simulink model "wlan_phy_tx_pmd"  (Simulink 7.8)
settings: Solver=VariableStepDiscrete  SolverMode=SingleTasking  StartTime=0.0  StopTime=inf  RelTol=1e-3
PostLoadFcn:
  | wlan_phy_tx_init
InitFcn:
  | wlan_phy_tx_init
StartFcn:
  | wlan_phy_tx_init
undefined symbols (not defined in the file): gcbh, ht_preamble_rom, MAX_CP_LEN, MAX_DATA_BITS_PER_SYM_PERIOD, MAX_NCBPS, MAX_NUM_BYTES, MAX_NUM_SC, MAX_NUM_SYMS, mcs_rom_11ag, mcs_rom_11n, Mod_Constellation_16QAM, Mod_Constellation_64QAM, Mod_Constellation_BPSK, Mod_Constellation_QPSK, Preamble_IQ, Preamble_IQ_scaled, tx_sim, wlan_tx_interleave_rom, xlBlockLoadCallback, xlGetNormalizedPeriod
libraries: xbsIndex_r4 x1358, xbsEDKLib_r4 x1
(part 6 of 10)

== system wlan_phy_tx_pmd/Start Ctrl/Simulation Stop ==
  TX_DONE : Inport
  Constant1 : Constant  Value=tx_sim.num_pkts
  Counter : xbsIndex_r4/Counter  cnt_type=Free Running  cnt_to=Inf  operation=Up  start_count=0  cnt_by_val=1  arith_type=Unsigned  n_bits=8  bin_pt=0  load_pin=off  rst=off  en=on  explicit_period=off  period=1  dbl_ovrd=off  use_behavioral_HDL=off  implementation=Fabric  block_type=counter
  Delay : xbsIndex_r4/Delay  rst=off  infoeditControl=Selection of Reset will increase slice count due to use of real FFs and instead of SRLs  en=off  latency=500  dbl_ovrd=off  reg_retiming=off  block_type=delay
  Delay1 : xbsIndex_r4/Delay  rst=off  infoeditControl=Selection of Reset will increase slice count due to use of real FFs and instead of SRLs  en=off  latency=32  dbl_ovrd=off  reg_retiming=off  block_type=delay
  Delay2 : Delay  DelayLength=400  SampleTime=1
  Disregard Subsystem : xbsIndex_r4/Disregard Subsystem  Tag=discardX  block_type=disregard
  Gateway Out{1..4} (4 alike) : xbsIndex_r4/Gateway Out  inherit_from_input=off  hdl_port=off  timing_constraint=None  locs_specified=off  LOCs={}  UseAsDAC=off  DACChannel='1'  block_type=gatewayout
  Posedge3 : Subsystem
  Radio TxEn-RxEn : Scope  NumInputPorts=7
      settings: TimeRange=14000  YMin=-1~2~-1~-1~-1~-1~-1  YMax=1~2~1~1~1~1~1  SaveName=ScopeData14
  Relational Operator : RelationalOperator  OutDataTypeStr=boolean
  S-R Latch1 : Subsystem
  Stop Simulation : Stop
  tag scope: sim_Start_New_Tx=global
  wires:
  Posedge3/1(Q) -> Counter/1, Delay/1
  Counter/1 -> Gateway Out1/1, Gateway Out4/1
  Constant1/1 -> Relational Operator/2
  Relational Operator/1 -> Delay2/1
  Gateway Out1/1 -> Relational Operator/1
  TX_DONE/1 -> Posedge3/1(D), Gateway Out3/1
  Delay2/1 -> Stop Simulation/1, Radio TxEn-RxEn/3  "Stop"
  S-R Latch1/1(Q) -> Delay1/1, Gateway Out2/1  "Start"
  Gateway Out3/1 -> Radio TxEn-RxEn/1  "TX_DONE"
  Gateway Out4/1 -> Radio TxEn-RxEn/2  "Pkt Count"
  Delay/1 -> S-R Latch1/1(S)
  Delay1/1 -> S-R Latch1/2(R)
  Gateway Out2/1 -> [sim_Start_New_Tx], Radio TxEn-RxEn/4  "Start"

== system wlan_phy_tx_pmd/Start Ctrl/Tx Active Debug Signal ==
  note: TX_RUNNING is a debug signal usually tied to an FPGA
      | output for real-time observation on an oscilloscope. The mux
      | here selects between the raw Tx Active signal or
      | a delayed version. The raw signal is useful for observing
      | MAC timing. The delayed version is useful for triggering
      | packet detection at an Rx node.
  Tx Active : Inport
  Convert9 : xbsIndex_r4/Convert  gui_display_data_type=Fixed-point  arith_type=Unsigned  n_bits=1  bin_pt=0  float_type=Single  exp_bits=8  fraction_bits=24  quantization=Truncate  overflow=Wrap  en=off  latency=0  dbl_ovrd=off  pipeline=off  block_type=convert
  Dly : Subsystem
  Mux : xbsIndex_r4/Mux  inputs=2  en=off  latency=0  precision=Full  arith_type=Unsigned  n_bits=16  bin_pt=14  quantization=Truncate  overflow=Wrap  dbl_ovrd=off  block_type=mux
  Register : xbsIndex_r4/Register  init=0  rst=off  en=off  dbl_ovrd=off  block_type=register
  Register1 : xbsIndex_r4/Register  init=0  rst=off  en=off  dbl_ovrd=off  block_type=register
  Register5 : xbsIndex_r4/Register  init=0  rst=off  en=off  dbl_ovrd=off  block_type=register
  dbg_TX_RUNNING : xbsIndex_r4/Gateway Out  inherit_from_input=off  hdl_port=on  timing_constraint=None  locs_specified=off  LOCs={}  UseAsDAC=off  DACChannel='1'  block_type=gatewayout
  wires:
  Register/1 -> Register1/1
  Register1/1 -> dbg_TX_RUNNING/1
  Dly/1(Q) -> Mux/3
  [regTx_TxRunning_Output_Sel] -> Mux/1
  Mux/1 -> Register/1
  Register5/1 -> Dly/1(D), Convert9/1
  Convert9/1 -> Mux/2
  Tx Active/1 -> Register5/1

== system wlan_phy_tx_pmd/Start Ctrl/Tx Gain ==
  note: Pass through MAC Tx gain setting to radio controller
  Sw Tx : Inport
  Hw Tx : Inport  Port=2
  Convert : xbsIndex_r4/Convert  gui_display_data_type=Boolean  arith_type=Boolean  n_bits=16  bin_pt=14  float_type=Single  exp_bits=8  fraction_bits=24  quantization=Truncate  overflow=Wrap  en=off  latency=0  dbl_ovrd=off  pipeline=off  block_type=convert
  Convert1 : xbsIndex_r4/Convert  gui_display_data_type=Boolean  arith_type=Boolean  n_bits=16  bin_pt=14  float_type=Single  exp_bits=8  fraction_bits=24  quantization=Truncate  overflow=Wrap  en=off  latency=0  dbl_ovrd=off  pipeline=off  block_type=convert
  Logical1 : xbsIndex_r4/Logical  logical_function=OR  inputs=2  en=off  latency=0  precision=Full  arith_type=Unsigned  n_bits=16  bin_pt=0  align_bp=on  dbl_ovrd=off  block_type=logical
  PHY_TX_GAIN_A : xbsIndex_r4/Gateway In  gui_display_data_type=Fixed-point  arith_type=Unsigned  n_bits=6  bin_pt=0  preci_type=Single  exp_width=8  frac_width=24  quantization="Round  (unbiased: +/- Inf)"  overflow=Saturate  period=1  dbl_ovrd=off  timing_constraint=None  locs_specified=off  LOCs={}  UseAsADC=off  ADCChannel='1'  inherit_from_input=off  hdl_port=on  block_type=gatewayin
  PHY_TX_GAIN_B : xbsIndex_r4/Gateway In  gui_display_data_type=Fixed-point  arith_type=Unsigned  n_bits=6  bin_pt=0  preci_type=Single  exp_width=8  frac_width=24  quantization="Round  (unbiased: +/- Inf)"  overflow=Saturate  period=1  dbl_ovrd=off  timing_constraint=None  locs_specified=off  LOCs={}  UseAsADC=off  ADCChannel='1'  inherit_from_input=off  hdl_port=on  block_type=gatewayin
  PHY_TX_GAIN_C : xbsIndex_r4/Gateway In  gui_display_data_type=Fixed-point  arith_type=Unsigned  n_bits=6  bin_pt=0  preci_type=Single  exp_width=8  frac_width=24  quantization="Round  (unbiased: +/- Inf)"  overflow=Saturate  period=1  dbl_ovrd=off  timing_constraint=None  locs_specified=off  LOCs={}  UseAsADC=off  ADCChannel='1'  inherit_from_input=off  hdl_port=on  block_type=gatewayin
  PHY_TX_GAIN_D : xbsIndex_r4/Gateway In  gui_display_data_type=Fixed-point  arith_type=Unsigned  n_bits=6  bin_pt=0  preci_type=Single  exp_width=8  frac_width=24  quantization="Round  (unbiased: +/- Inf)"  overflow=Saturate  period=1  dbl_ovrd=off  timing_constraint=None  locs_specified=off  LOCs={}  UseAsADC=off  ADCChannel='1'  inherit_from_input=off  hdl_port=on  block_type=gatewayin
  Register{1,3,5,7} (4 alike) : xbsIndex_r4/Register  init=0  rst=off  en=off  dbl_ovrd=off  block_type=register
  Register{2,4,6,8} (4 alike) : xbsIndex_r4/Register  init=0  rst=off  en=on  dbl_ovrd=off  block_type=register
      settings: xl_area=[1 1 0 0 0 0 0]  block_version=VER_STRING_GOES_HERE
  Tx Gain A : Outport
  Tx Gain B : Outport  Port=2
  Tx Gain C : Outport  Port=3
  Tx Gain D : Outport  Port=4
  wires:
  Convert1/1 -> Logical1/2
  Hw Tx/1 -> Convert1/1
  Sw Tx/1 -> Convert/1
  PHY_TX_GAIN_A/1 -> Register2/1
  Convert/1 -> Logical1/1
  Register2/1 -> Register1/1
  Logical1/1 -> Register2/2, Register4/2, Register6/2, Register8/2
  Register1/1 -> Tx Gain A/1
  Register4/1 -> Register3/1
  Register3/1 -> Tx Gain B/1
  PHY_TX_GAIN_B/1 -> Register4/1
  Register6/1 -> Register5/1
  Register5/1 -> Tx Gain C/1
  Register8/1 -> Register7/1
  Register7/1 -> Tx Gain D/1
  PHY_TX_GAIN_C/1 -> Register6/1
  PHY_TX_GAIN_D/1 -> Register8/1

== system wlan_phy_tx_pmd/Start Ctrl/negedge ==
  D : Inport
  Delay : xbsIndex_r4/Delay  rst=off  infoeditControl=Selection of Reset will increase slice count due to use of real FFs and instead of SRLs  en=off  latency=1  dbl_ovrd=off  reg_retiming=off  block_type=delay
      settings: infoedit=Hardware notes: A delay line is a chain, each link of which is an SRL16 followed by a flip-flop. If register retiming is enabled, the delay line is a chain of flip-flops.  xl_area=[1 1 0 0 0 0 0]  block_version=VER_STRING_GOES_HERE
  Inverter : xbsIndex_r4/Inverter  en=off  latency=0  dbl_ovrd=off  block_type=inv
      settings: xl_area=[0 0 0 0 0 0 0]  block_version=VER_STRING_GOES_HERE
  Logical1 : xbsIndex_r4/Logical  logical_function=AND  inputs=2  en=off  latency=0  precision=Full  arith_type=Unsigned  n_bits=8  bin_pt=2  align_bp=on  dbl_ovrd=off  block_type=logical
      settings: xl_area=[1 0 0 1 0 0 0]  block_version=VER_STRING_GOES_HERE
  Q : Outport
  wires:
  D/1 -> Delay/1, Inverter/1
  Logical1/1 -> Q/1
  Delay/1 -> Logical1/1
  Inverter/1 -> Logical1/2

== system wlan_phy_tx_pmd/IFFT and Cyclic Prefix/Buffer and Cyclic Prefix/Control ==
  note: Hacky way to skip last cycle of counter. Avoids
      | having to compute SC+CP-1.
  tlast : Inport
  AddSub : xbsIndex_r4/AddSub  mode=Addition  use_carryin=off  use_carryout=off  en=off  latency=1  precision=Full  arith_type=Unsigned  n_bits=16  bin_pt=14  quantization=Truncate  overflow=Wrap  dbl_ovrd=off  use_behavioral_HDL=off  hw_selection=Fabric  pipelined=off  block_type=addsub
  Counter : xbsIndex_r4/Counter  cnt_type=Free Running  cnt_to=47  operation=Up  start_count=0  cnt_by_val=1  arith_type=Unsigned  n_bits=ceil(log2(MAX_NUM_SC + MAX_CP_LEN) + 1)  bin_pt=0  load_pin=off  rst=on  en=on  explicit_period=off  period=1  dbl_ovrd=off  use_behavioral_HDL=off  implementation=Fabric  block_type=counter
  Inverter1 : xbsIndex_r4/Inverter  en=off  latency=0  dbl_ovrd=off  block_type=inv
      settings: xl_area=[0 0 0 0 0 0 0]  block_version=VER_STRING_GOES_HERE
  Inverter2 : xbsIndex_r4/Inverter  en=off  latency=0  dbl_ovrd=off  block_type=inv
      settings: xl_area=[0 0 0 0 0 0 0]  block_version=VER_STRING_GOES_HERE
  Logical2 : xbsIndex_r4/Logical  logical_function=AND  inputs=2  en=off  latency=0  precision=Full  arith_type=Unsigned  n_bits=16  bin_pt=0  align_bp=on  dbl_ovrd=off  block_type=logical
  Relational3 : xbsIndex_r4/Relational  mode=a>=b  en=off  latency=0  dbl_ovrd=off  block_type=relational
  S-R Latch1 : Subsystem
  Rd Addr : Outport
  Valid : Outport  Port=2
  wires:
  [regTx_NUM_SC] -> AddSub/1
  Inverter1/1 -> Counter/1
  S-R Latch1/1(Q) -> Counter/2, Inverter1/1, Logical2/1
  Counter/1 -> Relational3/1, Rd Addr/1
  [regTx_CP_LEN] -> AddSub/2
  Relational3/1 -> S-R Latch1/2(R), Inverter2/1
  Inverter2/1 -> Logical2/2
  tlast/1 -> S-R Latch1/1(S)
  Logical2/1 -> Valid/1
  AddSub/1 -> Relational3/2

== system wlan_phy_tx_pmd/IFFT and Cyclic Prefix/Buffer and Cyclic Prefix/I/Q Concat ==
  I : Inport
  Q : Inport  Port=2
  Concat : xbsIndex_r4/Concat  num_inputs=2  dbl_ovrd=off  block_type=concat
  Reinterpret : xbsIndex_r4/Reinterpret  force_arith_type=on  arith_type=Unsigned  force_bin_pt=on  bin_pt=0  block_type=reinterpret
  Reinterpret1 : xbsIndex_r4/Reinterpret  force_arith_type=on  arith_type=Unsigned  force_bin_pt=on  bin_pt=0  block_type=reinterpret
  IQ : Outport
  wires:
  Reinterpret/1 -> Concat/1
  Reinterpret1/1 -> Concat/2
  I/1 -> Reinterpret/1
  Concat/1 -> IQ/1
  Q/1 -> Reinterpret1/1

== system wlan_phy_tx_pmd/IFFT and Cyclic Prefix/Buffer and Cyclic Prefix/I/Q Slice ==
  IQ : Inport
  Reinterpret2 : xbsIndex_r4/Reinterpret  force_arith_type=on  arith_type="Signed  (2's comp)"  force_bin_pt=on  bin_pt=15  block_type=reinterpret
  Reinterpret3 : xbsIndex_r4/Reinterpret  force_arith_type=on  arith_type="Signed  (2's comp)"  force_bin_pt=on  bin_pt=15  block_type=reinterpret
  Slice : xbsIndex_r4/Slice  nbits=16  boolean_output=off  mode=Upper Bit Location + Width  bit1=0  base1=MSB of Input  bit0=0  base0=LSB of Input  dbl_ovrd=off  block_type=slice
  Slice1 : xbsIndex_r4/Slice  nbits=16  boolean_output=off  mode=Lower Bit Location + Width  bit1=0  base1=MSB of Input  bit0=0  base0=LSB of Input  dbl_ovrd=off  block_type=slice
  I : Outport
  Q : Outport  Port=2
  wires:
  Reinterpret3/1 -> Q/1
  Reinterpret2/1 -> I/1
  IQ/1 -> Slice/1, Slice1/1
  Slice1/1 -> Reinterpret3/1
  Slice/1 -> Reinterpret2/1

== system wlan_phy_tx_pmd/IFFT and Cyclic Prefix/FIFO/I/Q Concat ==
  I : Inport
  Q : Inport  Port=2
  Concat : xbsIndex_r4/Concat  num_inputs=2  dbl_ovrd=off  block_type=concat
  Reinterpret : xbsIndex_r4/Reinterpret  force_arith_type=on  arith_type=Unsigned  force_bin_pt=on  bin_pt=0  block_type=reinterpret
  Reinterpret1 : xbsIndex_r4/Reinterpret  force_arith_type=on  arith_type=Unsigned  force_bin_pt=on  bin_pt=0  block_type=reinterpret
  IQ : Outport
  wires:
  Reinterpret/1 -> Concat/1
  Reinterpret1/1 -> Concat/2
  I/1 -> Reinterpret/1
  Concat/1 -> IQ/1
  Q/1 -> Reinterpret1/1

== system wlan_phy_tx_pmd/IFFT and Cyclic Prefix/FIFO/I/Q Slice ==
  IQ : Inport
  Reinterpret2 : xbsIndex_r4/Reinterpret  force_arith_type=on  arith_type="Signed  (2's comp)"  force_bin_pt=on  bin_pt=15  block_type=reinterpret
  Reinterpret3 : xbsIndex_r4/Reinterpret  force_arith_type=on  arith_type="Signed  (2's comp)"  force_bin_pt=on  bin_pt=15  block_type=reinterpret
  Slice : xbsIndex_r4/Slice  nbits=16  boolean_output=off  mode=Upper Bit Location + Width  bit1=0  base1=MSB of Input  bit0=0  base0=LSB of Input  dbl_ovrd=off  block_type=slice
  Slice1 : xbsIndex_r4/Slice  nbits=16  boolean_output=off  mode=Lower Bit Location + Width  bit1=0  base1=MSB of Input  bit0=0  base0=LSB of Input  dbl_ovrd=off  block_type=slice
  I : Outport
  Q : Outport  Port=2
  wires:
  Reinterpret3/1 -> Q/1
  Reinterpret2/1 -> I/1
  IQ/1 -> Slice/1, Slice1/1
  Slice1/1 -> Reinterpret3/1
  Slice/1 -> Reinterpret2/1

== system wlan_phy_tx_pmd/OFDM Symbol Ctrl/Sym Counter/S-R Latch1 ==
  S : Inport
  R : Inport  Port=2
  Constant1 : xbsIndex_r4/Constant  const=1  gui_display_data_type=Fixed-point  arith_type=Boolean  n_bits=1  bin_pt=0  preci_type=Single  exp_width=8  frac_width=24  explicit_period=off  period=1  equ=P=C  opselect=C  inp2=PCIN>>17  opr=+  inp1=P  carry=CIN  dbl_ovrd=off  block_type=constant
      settings: block_version=VER_STRING_GOES_HERE
  Convert1 : xbsIndex_r4/Convert  gui_display_data_type=Boolean  arith_type=Boolean  n_bits=1  bin_pt=0  float_type=Single  exp_bits=8  fraction_bits=24  quantization=Truncate  overflow=Wrap  en=off  latency=0  dbl_ovrd=off  pipeline=off  block_type=convert
  Convert2 : xbsIndex_r4/Convert  gui_display_data_type=Boolean  arith_type=Boolean  n_bits=1  bin_pt=0  float_type=Single  exp_bits=8  fraction_bits=24  quantization=Truncate  overflow=Wrap  en=off  latency=0  dbl_ovrd=off  pipeline=off  block_type=convert
  Register2 : xbsIndex_r4/Register  init=0  rst=on  en=on  dbl_ovrd=off  block_type=register
      settings: xl_area=[1 1 0 0 0 0 0]  block_version=VER_STRING_GOES_HERE
  Q : Outport
  wires:
  Convert2/1 -> Register2/3
  Convert1/1 -> Register2/2
  Constant1/1 -> Register2/1
  R/1 -> Convert1/1
  Register2/1 -> Q/1
  S/1 -> Convert2/1

== system wlan_phy_tx_pmd/OFDM Symbol Ctrl/Sym Samp Counter/Posedge1 ==
  D : Inport
  Delay : xbsIndex_r4/Delay  rst=off  infoeditControl=Selection of Reset will increase slice count due to use of real FFs and instead of SRLs  en=off  latency=1  dbl_ovrd=off  reg_retiming=off  block_type=delay
      settings: infoedit=Hardware notes: A delay line is a chain, each link of which is an SRL16 followed by a flip-flop. If register retiming is enabled, the delay line is a chain of flip-flops.  xl_area=[1 1 0 0 0 0 0]  block_version=VER_STRING_GOES_HERE
  Inverter : xbsIndex_r4/Inverter  en=off  latency=0  dbl_ovrd=off  block_type=inv
      settings: xl_area=[0 0 0 0 0 0 0]  block_version=VER_STRING_GOES_HERE
  Logical1 : xbsIndex_r4/Logical  logical_function=AND  inputs=2  en=off  latency=0  precision=Full  arith_type=Unsigned  n_bits=8  bin_pt=2  align_bp=on  dbl_ovrd=off  block_type=logical
      settings: xl_area=[1 0 0 1 0 0 0]  block_version=VER_STRING_GOES_HERE
  Q : Outport
  wires:
  Inverter/1 -> Logical1/1
  D/1 -> Logical1/2, Delay/1
  Logical1/1 -> Q/1
  Delay/1 -> Inverter/1

== system wlan_phy_tx_pmd/OFDM Symbol Ctrl/Sym Samp Counter/Posedge2 ==
  D : Inport
  Delay : xbsIndex_r4/Delay  rst=off  infoeditControl=Selection of Reset will increase slice count due to use of real FFs and instead of SRLs  en=off  latency=1  dbl_ovrd=off  reg_retiming=off  block_type=delay
      settings: infoedit=Hardware notes: A delay line is a chain, each link of which is an SRL16 followed by a flip-flop. If register retiming is enabled, the delay line is a chain of flip-flops.  xl_area=[1 1 0 0 0 0 0]  block_version=VER_STRING_GOES_HERE
  Inverter : xbsIndex_r4/Inverter  en=off  latency=0  dbl_ovrd=off  block_type=inv
      settings: xl_area=[0 0 0 0 0 0 0]  block_version=VER_STRING_GOES_HERE
  Logical1 : xbsIndex_r4/Logical  logical_function=AND  inputs=2  en=off  latency=0  precision=Full  arith_type=Unsigned  n_bits=8  bin_pt=2  align_bp=on  dbl_ovrd=off  block_type=logical
      settings: xl_area=[1 0 0 1 0 0 0]  block_version=VER_STRING_GOES_HERE
  Q : Outport
  wires:
  Delay/1 -> Inverter/1
  Logical1/1 -> Q/1
  D/1 -> Delay/1, Logical1/2
  Inverter/1 -> Logical1/1

== system wlan_phy_tx_pmd/OFDM Symbol Ctrl/Sym Samp Counter/S-R Latch2 ==
  S : Inport
  R : Inport  Port=2
  Constant1 : xbsIndex_r4/Constant  const=1  gui_display_data_type=Fixed-point  arith_type=Boolean  n_bits=1  bin_pt=0  preci_type=Single  exp_width=8  frac_width=24  explicit_period=off  period=1  equ=P=C  opselect=C  inp2=PCIN>>17  opr=+  inp1=P  carry=CIN  dbl_ovrd=off  block_type=constant
      settings: block_version=VER_STRING_GOES_HERE
  Convert1 : xbsIndex_r4/Convert  gui_display_data_type=Boolean  arith_type=Boolean  n_bits=1  bin_pt=0  float_type=Single  exp_bits=8  fraction_bits=24  quantization=Truncate  overflow=Wrap  en=off  latency=0  dbl_ovrd=off  pipeline=off  block_type=convert
  Convert2 : xbsIndex_r4/Convert  gui_display_data_type=Boolean  arith_type=Boolean  n_bits=1  bin_pt=0  float_type=Single  exp_bits=8  fraction_bits=24  quantization=Truncate  overflow=Wrap  en=off  latency=0  dbl_ovrd=off  pipeline=off  block_type=convert
  Register2 : xbsIndex_r4/Register  init=0  rst=on  en=on  dbl_ovrd=off  block_type=register
      settings: xl_area=[1 1 0 0 0 0 0]  block_version=VER_STRING_GOES_HERE
  Q : Outport
  wires:
  S/1 -> Convert2/1
  Register2/1 -> Q/1
  R/1 -> Convert1/1
  Constant1/1 -> Register2/1
  Convert1/1 -> Register2/2
  Convert2/1 -> Register2/3

== system wlan_phy_tx_pmd/PSDU Syms Gen/Index Gen/Bit Index Gen ==
  Bit Rd En : Inport
  Bit counter : xbsIndex_r4/Counter  cnt_type=Free Running  cnt_to=6  operation=Up  start_count=0  cnt_by_val=1  arith_type=Unsigned  n_bits=ceil(log2(MAX_NUM_BYTES))+3  bin_pt=0  load_pin=off  rst=on  en=on  explicit_period=off  period=1  dbl_ovrd=off  use_behavioral_HDL=off  implementation=Fabric  block_type=counter
  Bit in Byte : xbsIndex_r4/Slice  nbits=3  boolean_output=off  mode=Lower Bit Location + Width  bit1=0  base1=MSB of Input  bit0=0  base0=LSB of Input  dbl_ovrd=off  block_type=slice
      settings: block_version=8.2.02
  Bytes : xbsIndex_r4/Slice  nbits=ceil(log2(MAX_NUM_BYTES))  boolean_output=off  mode=Upper Bit Location + Width  bit1=0  base1=MSB of Input  bit0=0  base0=LSB of Input  dbl_ovrd=off  block_type=slice
      settings: block_version=8.2.02
  Constant3 : xbsIndex_r4/Constant  const=0  gui_display_data_type=Fixed-point  arith_type=Unsigned  n_bits=2  bin_pt=0  preci_type=Single  exp_width=8  frac_width=24  explicit_period=off  period=1  equ=P=C  opselect=C  inp2=PCIN>>17  opr=+  inp1=P  carry=CIN  dbl_ovrd=off  block_type=constant
      settings: block_version=VER_STRING_GOES_HERE
  Logical5 : xbsIndex_r4/Logical  logical_function=AND  inputs=2  en=off  latency=0  precision=Full  arith_type=Unsigned  n_bits=16  bin_pt=0  align_bp=on  dbl_ovrd=off  block_type=logical
  Relational1 : xbsIndex_r4/Relational  mode=a=b  en=off  latency=0  dbl_ovrd=off  block_type=relational
  Byte Ind : Outport
  Byte Ind Valid : Outport  Port=2
  Bit Sel : Outport  Port=3
  Bit Sel Valid : Outport  Port=4
  wires:
  Bit counter/1 -> Bytes/1, Bit in Byte/1
  Bit in Byte/1 -> Bit Sel/1, Relational1/1
  Bytes/1 -> Byte Ind/1
  Constant3/1 -> Relational1/2
  Relational1/1 -> Logical5/1
  Logical5/1 -> Byte Ind Valid/1
  Bit Rd En/1 -> Logical5/2, Bit Sel Valid/1, Bit counter/2
  [TX_RESET] -> Bit counter/1

== system wlan_phy_tx_pmd/PSDU Syms Gen/Index Gen/Bits Per Sym ==
  note: SIGNAL and HT-SIG sybmols always
      | contain 24 data bits (48 subcarriers, BPSK, 1/2 rate)
      | This mux selects the N_DBPS value for the current
      | MCS sometime after the SIGNAL (11a) or HT-SIG (11n)
      | fields are decoded.
      | Initial vlaue of N_DBPS register at mux in 0 must be non-zero!
  note: This block asserts the "Bit Rd En" output for a number of cycles
      | equal to the number of bits that will be read from the packet
      | buffer. Each OFDM symbol contains either 24 bits (for PHY
      | preamble symbols) or DATA_N_DBPS bits (set by the packet's MCS).
  Start : Inport
  Base Rate : Inport  Port=2
  Full Rate : Inport  Port=3
  Constant2 : xbsIndex_r4/Constant  const=24  gui_display_data_type=Fixed-point  arith_type=Unsigned  n_bits=5  bin_pt=0  preci_type=Single  exp_width=8  frac_width=24  explicit_period=off  period=1  equ=P=C  opselect=C  inp2=PCIN>>17  opr=+  inp1=P  carry=CIN  dbl_ovrd=off  block_type=constant
  Counter : xbsIndex_r4/Counter  cnt_type=Free Running  cnt_to=47  operation=Up  start_count=0  cnt_by_val=1  arith_type=Unsigned  n_bits=ceil(log2(MAX_DATA_BITS_PER_SYM_PERIOD))  bin_pt=0  load_pin=off  rst=on  en=on  explicit_period=off  period=1  dbl_ovrd=off  use_behavioral_HDL=off  implementation=Fabric  block_type=counter
  Inverter : xbsIndex_r4/Inverter  en=off  latency=0  dbl_ovrd=off  block_type=inv
      settings: xl_area=[0 0 0 0 0 0 0]  block_version=VER_STRING_GOES_HERE
  Inverter1 : xbsIndex_r4/Inverter  en=off  latency=0  dbl_ovrd=off  block_type=inv
      settings: xl_area=[0 0 0 0 0 0 0]  block_version=VER_STRING_GOES_HERE
  Logical1 : xbsIndex_r4/Logical  logical_function=OR  inputs=2  en=off  latency=0  precision=Full  arith_type=Unsigned  n_bits=8  bin_pt=2  align_bp=on  dbl_ovrd=off  block_type=logical
      settings: xl_area=[1 0 0 1 0 0 0]  block_version=VER_STRING_GOES_HERE
  Logical2 : xbsIndex_r4/Logical  logical_function=OR  inputs=2  en=off  latency=0  precision=Full  arith_type=Unsigned  n_bits=8  bin_pt=2  align_bp=on  dbl_ovrd=off  block_type=logical
      settings: xl_area=[1 0 0 1 0 0 0]  block_version=VER_STRING_GOES_HERE
  Logical3 : xbsIndex_r4/Logical  logical_function=AND  inputs=2  en=off  latency=0  precision=Full  arith_type=Unsigned  n_bits=8  bin_pt=2  align_bp=on  dbl_ovrd=off  block_type=logical
      settings: xl_area=[1 0 0 1 0 0 0]  block_version=VER_STRING_GOES_HERE
  Logical4 : xbsIndex_r4/Logical  logical_function=AND  inputs=2  en=off  latency=0  precision=Full  arith_type=Unsigned  n_bits=8  bin_pt=2  align_bp=on  dbl_ovrd=off  block_type=logical
      settings: xl_area=[1 0 0 1 0 0 0]  block_version=VER_STRING_GOES_HERE
  Mux : xbsIndex_r4/Mux  inputs=2  en=off  latency=0  precision=Full  arith_type=Unsigned  n_bits=16  bin_pt=14  quantization=Truncate  overflow=Wrap  dbl_ovrd=off  block_type=mux
  Register2 : xbsIndex_r4/Register  init=24  rst=on  en=on  dbl_ovrd=off  block_type=register
      settings: xl_area=[1 1 0 0 0 0 0]  block_version=VER_STRING_GOES_HERE
  Register3 : xbsIndex_r4/Register  init=0  rst=on  en=on  dbl_ovrd=off  block_type=register
      settings: xl_area=[1 1 0 0 0 0 0]  block_version=VER_STRING_GOES_HERE
  Relational3 : xbsIndex_r4/Relational  mode=a<b  en=off  latency=0  dbl_ovrd=off  block_type=relational
  S-R Latch1 : Subsystem
  Rd En : Outport
  wires:
  Logical2/1 -> Logical3/2
  Constant2/1 -> Mux/3
  Register2/1 -> Mux/2
  Register3/1 -> Mux/1
  [TX_RESET] -> Register3/2, Register2/2
  Inverter/1 -> Logical1/2
  Logical1/1 -> S-R Latch1/2(R)
  [TX_RESET] -> Logical1/1
  [OFDM_TX_DATA_N_DBPS] -> Register2/1
  Inverter1/1 -> Counter/1
  Relational3/1 -> Logical4/1, Inverter/1
  Mux/1 -> Relational3/2
  Counter/1 -> Relational3/1
  Logical3/1 -> Register3/3, Register2/3, S-R Latch1/1(S)
  S-R Latch1/1(Q) -> Logical4/2, Inverter1/1, Counter/2
  Logical4/1 -> Rd En/1
  Start/1 -> Logical3/1
  Base Rate/1 -> Logical2/2, Register3/1
  Full Rate/1 -> Logical2/1

== system wlan_phy_tx_pmd/PSDU Syms Gen/Modulate/16QAM Mod ==
  note: 16-QAM Bit Mapping:
      | [b0 b1] / [b2 b3]:
      | 00 = -3
      | 01 = -1
      | 11 = +1
      | 10 = +3
      | Norm = 1/sqrt(10)
  note: 00 -> 00
  note: 10 -> 01
  note: 01 -> 10
  note: 11 -> 11
  b[3:0] : Inport
  Constant1 : xbsIndex_r4/Constant  const=Mod_Constellation_16QAM(3)  gui_display_data_type=Fixed-point  arith_type=Signed (2's comp)  n_bits=12  bin_pt=11  preci_type=Single  exp_width=8  frac_width=24  explicit_period=off  period=1  equ=P=C  opselect=C  inp2=PCIN>>17  opr=+  inp1=P  carry=CIN  dbl_ovrd=off  block_type=constant
  Constant2 : xbsIndex_r4/Constant  const=Mod_Constellation_16QAM(1)  gui_display_data_type=Fixed-point  arith_type=Signed (2's comp)  n_bits=12  bin_pt=11  preci_type=Single  exp_width=8  frac_width=24  explicit_period=off  period=1  equ=P=C  opselect=C  inp2=PCIN>>17  opr=+  inp1=P  carry=CIN  dbl_ovrd=off  block_type=constant
  Constant3 : xbsIndex_r4/Constant  const=Mod_Constellation_16QAM(2)  gui_display_data_type=Fixed-point  arith_type=Signed (2's comp)  n_bits=12  bin_pt=11  preci_type=Single  exp_width=8  frac_width=24  explicit_period=off  period=1  equ=P=C  opselect=C  inp2=PCIN>>17  opr=+  inp1=P  carry=CIN  dbl_ovrd=off  block_type=constant
  Constant4 : xbsIndex_r4/Constant  const=Mod_Constellation_16QAM(4)  gui_display_data_type=Fixed-point  arith_type=Signed (2's comp)  n_bits=12  bin_pt=11  preci_type=Single  exp_width=8  frac_width=24  explicit_period=off  period=1  equ=P=C  opselect=C  inp2=PCIN>>17  opr=+  inp1=P  carry=CIN  dbl_ovrd=off  block_type=constant
  Mux : xbsIndex_r4/Mux  inputs=4  en=off  latency=0  precision=Full  arith_type=Unsigned  n_bits=16  bin_pt=14  quantization=Truncate  overflow=Wrap  dbl_ovrd=off  block_type=mux
  Mux1 : xbsIndex_r4/Mux  inputs=4  en=off  latency=0  precision=Full  arith_type=Unsigned  n_bits=16  bin_pt=14  quantization=Truncate  overflow=Wrap  dbl_ovrd=off  block_type=mux
  b[1:0] : xbsIndex_r4/Slice  nbits=2  boolean_output=off  mode=Lower Bit Location + Width  bit1=0  base1=MSB of Input  bit0=0  base0=LSB of Input  dbl_ovrd=off  block_type=slice
  b[3:2] : xbsIndex_r4/Slice  nbits=2  boolean_output=off  mode=Lower Bit Location + Width  bit1=0  base1=MSB of Input  bit0=2  base0=LSB of Input  dbl_ovrd=off  block_type=slice
  I : Outport
  Q : Outport  Port=2
  wires:
  b[1:0]/1 -> Mux/1
  b[3:0]/1 -> b[1:0]/1, b[3:2]/1
  Constant2/1 -> Mux/2, Mux1/2
  Constant1/1 -> Mux/3, Mux1/3
  Constant3/1 -> Mux/4, Mux1/4
  Constant4/1 -> Mux/5, Mux1/5
  b[3:2]/1 -> Mux1/1
  Mux/1 -> I/1
  Mux1/1 -> Q/1

== system wlan_phy_tx_pmd/PSDU Syms Gen/Modulate/64QAM Mod ==
  note: 64-QAM Bit Mapping:
      | [b0 b1 b2] / [b3 b4 b5]:
      | 000 = -7
      | 001 = -5
      | 010 = -1
      | 011 = -3
      | 100 = +7
      | 101 = +5
      | 110 = +1
      | 111 = +3
      |
      | Norm = 1/sqrt(42)
  note: Endian swap here - mux sels are [b2 b1 b0] and [b5 b4 b3]
  note: 000
  note: 001
  note: 010
  note: 011
  note: 100
  note: 101
  note: 110
  note: 111
  b[5:0] : Inport
  Constant1 : xbsIndex_r4/Constant  const=Mod_Constellation_64QAM(5)  gui_display_data_type=Fixed-point  arith_type=Signed (2's comp)  n_bits=12  bin_pt=11  preci_type=Single  exp_width=8  frac_width=24  explicit_period=off  period=1  equ=P=C  opselect=C  inp2=PCIN>>17  opr=+  inp1=P  carry=CIN  dbl_ovrd=off  block_type=constant
  Constant10 : xbsIndex_r4/Constant  const=Mod_Constellation_64QAM(2)  gui_display_data_type=Fixed-point  arith_type=Signed (2's comp)  n_bits=12  bin_pt=11  preci_type=Single  exp_width=8  frac_width=24  explicit_period=off  period=1  equ=P=C  opselect=C  inp2=PCIN>>17  opr=+  inp1=P  carry=CIN  dbl_ovrd=off  block_type=constant
  Constant11 : xbsIndex_r4/Constant  const=Mod_Constellation_64QAM(4)  gui_display_data_type=Fixed-point  arith_type=Signed (2's comp)  n_bits=12  bin_pt=11  preci_type=Single  exp_width=8  frac_width=24  explicit_period=off  period=1  equ=P=C  opselect=C  inp2=PCIN>>17  opr=+  inp1=P  carry=CIN  dbl_ovrd=off  block_type=constant
  Constant12 : xbsIndex_r4/Constant  const=Mod_Constellation_64QAM(8)  gui_display_data_type=Fixed-point  arith_type=Signed (2's comp)  n_bits=12  bin_pt=11  preci_type=Single  exp_width=8  frac_width=24  explicit_period=off  period=1  equ=P=C  opselect=C  inp2=PCIN>>17  opr=+  inp1=P  carry=CIN  dbl_ovrd=off  block_type=constant
  Constant2 : xbsIndex_r4/Constant  const=Mod_Constellation_64QAM(1)  gui_display_data_type=Fixed-point  arith_type=Signed (2's comp)  n_bits=12  bin_pt=11  preci_type=Single  exp_width=8  frac_width=24  explicit_period=off  period=1  equ=P=C  opselect=C  inp2=PCIN>>17  opr=+  inp1=P  carry=CIN  dbl_ovrd=off  block_type=constant
  Constant3 : xbsIndex_r4/Constant  const=Mod_Constellation_64QAM(3)  gui_display_data_type=Fixed-point  arith_type=Signed (2's comp)  n_bits=12  bin_pt=11  preci_type=Single  exp_width=8  frac_width=24  explicit_period=off  period=1  equ=P=C  opselect=C  inp2=PCIN>>17  opr=+  inp1=P  carry=CIN  dbl_ovrd=off  block_type=constant
  Constant4 : xbsIndex_r4/Constant  const=Mod_Constellation_64QAM(7)  gui_display_data_type=Fixed-point  arith_type=Signed (2's comp)  n_bits=12  bin_pt=11  preci_type=Single  exp_width=8  frac_width=24  explicit_period=off  period=1  equ=P=C  opselect=C  inp2=PCIN>>17  opr=+  inp1=P  carry=CIN  dbl_ovrd=off  block_type=constant
  Constant9 : xbsIndex_r4/Constant  const=Mod_Constellation_64QAM(6)  gui_display_data_type=Fixed-point  arith_type=Signed (2's comp)  n_bits=12  bin_pt=11  preci_type=Single  exp_width=8  frac_width=24  explicit_period=off  period=1  equ=P=C  opselect=C  inp2=PCIN>>17  opr=+  inp1=P  carry=CIN  dbl_ovrd=off  block_type=constant
  Mux : xbsIndex_r4/Mux  inputs=8  en=off  latency=0  precision=Full  arith_type=Unsigned  n_bits=16  bin_pt=14  quantization=Truncate  overflow=Wrap  dbl_ovrd=off  block_type=mux
  Mux1 : xbsIndex_r4/Mux  inputs=8  en=off  latency=0  precision=Full  arith_type=Unsigned  n_bits=16  bin_pt=14  quantization=Truncate  overflow=Wrap  dbl_ovrd=off  block_type=mux
  b[2:0] : xbsIndex_r4/Slice  nbits=3  boolean_output=off  mode=Lower Bit Location + Width  bit1=0  base1=MSB of Input  bit0=0  base0=LSB of Input  dbl_ovrd=off  block_type=slice
  b[5:3] : xbsIndex_r4/Slice  nbits=3  boolean_output=off  mode=Lower Bit Location + Width  bit1=0  base1=MSB of Input  bit0=3  base0=LSB of Input  dbl_ovrd=off  block_type=slice
  I : Outport
  Q : Outport  Port=2
  wires:
  Constant4/1 -> Mux/5, Mux1/5
  Constant3/1 -> Mux/4, Mux1/4
  Constant1/1 -> Mux/3, Mux1/3
  Constant2/1 -> Mux/2, Mux1/2
  b[5:0]/1 -> b[5:3]/1, b[2:0]/1
  b[2:0]/1 -> Mux/1
  Constant10/1 -> Mux/6, Mux1/6
  Constant9/1 -> Mux/7, Mux1/7
  Constant11/1 -> Mux/8, Mux1/8
  Constant12/1 -> Mux/9, Mux1/9
  Mux/1 -> I/1
  b[5:3]/1 -> Mux1/1
  Mux1/1 -> Q/1

== system wlan_phy_tx_pmd/PSDU Syms Gen/Modulate/BPSK Mod ==
  b[0] : Inport
  rot : Inport  Port=2
  Constant2 : xbsIndex_r4/Constant  const=Mod_Constellation_BPSK(1)  gui_display_data_type=Fixed-point  arith_type=Signed (2's comp)  n_bits=12  bin_pt=11  preci_type=Single  exp_width=8  frac_width=24  explicit_period=off  period=1  equ=P=C  opselect=C  inp2=PCIN>>17  opr=+  inp1=P  carry=CIN  dbl_ovrd=off  block_type=constant
  Constant3 : xbsIndex_r4/Constant  const=Mod_Constellation_BPSK(2)  gui_display_data_type=Fixed-point  arith_type=Signed (2's comp)  n_bits=12  bin_pt=11  preci_type=Single  exp_width=8  frac_width=24  explicit_period=off  period=1  equ=P=C  opselect=C  inp2=PCIN>>17  opr=+  inp1=P  carry=CIN  dbl_ovrd=off  block_type=constant
  Constant4 : xbsIndex_r4/Constant  const=0  gui_display_data_type=Fixed-point  arith_type=Signed (2's comp)  n_bits=12  bin_pt=11  preci_type=Single  exp_width=8  frac_width=24  explicit_period=off  period=1  equ=P=C  opselect=C  inp2=PCIN>>17  opr=+  inp1=P  carry=CIN  dbl_ovrd=off  block_type=constant
  Mux : xbsIndex_r4/Mux  inputs=2  en=off  latency=0  precision=Full  arith_type=Unsigned  n_bits=16  bin_pt=14  quantization=Truncate  overflow=Wrap  dbl_ovrd=off  block_type=mux
  Mux1 : xbsIndex_r4/Mux  inputs=2  en=off  latency=0  precision=Full  arith_type=Unsigned  n_bits=16  bin_pt=14  quantization=Truncate  overflow=Wrap  dbl_ovrd=off  block_type=mux
  Mux2 : xbsIndex_r4/Mux  inputs=2  en=off  latency=0  precision=Full  arith_type=Unsigned  n_bits=16  bin_pt=14  quantization=Truncate  overflow=Wrap  dbl_ovrd=off  block_type=mux
  I : Outport
  Q : Outport  Port=2
  wires:
  Mux/1 -> Mux1/2, Mux2/3
  Constant3/1 -> Mux/3
  Constant2/1 -> Mux/2
  b[0]/1 -> Mux/1
  rot/1 -> Mux1/1, Mux2/1
  Mux1/1 -> I/1
  Constant4/1 -> Mux1/3, Mux2/2
  Mux2/1 -> Q/1

== system wlan_phy_tx_pmd/PSDU Syms Gen/Modulate/Control & Pilots ==
  note: 1 cycle for RAM access
  Full Rate : Inport
  Pilot Shift : Inport  Port=2
  Sym Bits Rdy : Inport  Port=3
  IQ FIFO tready : Inport  Port=4
  Concat1 : xbsIndex_r4/Concat  num_inputs=2  dbl_ovrd=off  block_type=concat
  Data SC Map : Subsystem
  Delay{,1..2,5..6} (5 alike) : xbsIndex_r4/Delay  rst=off  infoeditControl=Selection of Reset will increase slice count due to use of real FFs and instead of SRLs  en=off  latency=1  dbl_ovrd=off  reg_retiming=off  block_type=delay
  Gateway Out{1..8} (8 alike) : xbsIndex_r4/Gateway Out  inherit_from_input=off  hdl_port=off  timing_constraint=None  locs_specified=off  LOCs={}  UseAsDAC=off  DACChannel='1'  block_type=gatewayout
  Logical : xbsIndex_r4/Logical  logical_function=OR  inputs=2  en=off  latency=0  precision=Full  arith_type=Unsigned  n_bits=8  bin_pt=2  align_bp=on  dbl_ovrd=off  block_type=logical
      settings: xl_area=[0, 0, 0, 0, 0, 0, 0]  block_version=VER_STRING_GOES_HERE
  Logical1 : xbsIndex_r4/Logical  logical_function=AND  inputs=2  en=off  latency=0  precision=Full  arith_type=Unsigned  n_bits=8  bin_pt=2  align_bp=on  dbl_ovrd=off  block_type=logical
      settings: xl_area=[0, 0, 0, 0, 0, 0, 0]  block_version=VER_STRING_GOES_HERE
  Mod Ctrl : Scope  NumInputPorts=8
      settings: TimeRange=8000  YMin=0~0~0~0~0~0~0~-1  YMax=1~1~1~60~80~2~1~1  SaveName=ScopeData4
  Pilot Gen : Subsystem
  Posedge : Subsystem
  Posedge1 : Subsystem
  S-R Latch1 : Subsystem
  Subcarrier Index Count : Subsystem
  Pilot I : Outport
  IQ Sel : Outport  Port=2
  IQ tvalid : Outport  Port=3
  IQ tlast : Outport  Port=4
  Data Sym Ind : Outport  Port=5
  wires:
  Subcarrier Index Count/1(sc_ind) -> Data SC Map/2(sc_ind), Pilot Gen/1(sc_ind), Gateway Out4/1
  Pilot Gen/1(pilot_valid) -> Concat1/2
  Data SC Map/2(data_sym_valid) -> Concat1/1
  Data SC Map/1(data_sym_ind) -> Data Sym Ind/1, Delay2/1
  Concat1/1 -> Delay5/1
  Pilot Gen/2(Pilot_I) -> Delay6/1
  [TX_RESET] -> Subcarrier Index Count/2(reset), Pilot Gen/2(reset), Logical/1
  Sym Bits Rdy/1 -> Posedge/1(D), Gateway Out8/1
  Posedge/1(Q) -> S-R Latch1/1(S)
  Subcarrier Index Count/2(last) -> Logical/2, Delay1/1
  Posedge1/1(Q) -> S-R Latch1/2(R)
  Logical/1 -> Posedge1/1(D)
  S-R Latch1/1(Q) -> Delay/1, Logical1/1
  Delay/1 -> IQ tvalid/1, Gateway Out1/1
  Delay1/1 -> IQ tlast/1, Gateway Out2/1
  Gateway Out8/1 -> Mod Ctrl/1  "Sym Bits Ready"
  Gateway Out1/1 -> Mod Ctrl/2  "IQ tvalid"
  Gateway Out2/1 -> Mod Ctrl/3  "IQ tlast"
  Gateway Out3/1 -> Mod Ctrl/4  "Data Sym Ind"
  Delay5/1 -> IQ Sel/1, Gateway Out5/1
  Delay6/1 -> Pilot I/1, Gateway Out7/1
  Logical1/1 -> Subcarrier Index Count/1(en)
  IQ FIFO tready/1 -> Logical1/2
  Gateway Out4/1 -> Mod Ctrl/5  "Sc Ind"
  Full Rate/1 -> Data SC Map/1(Full Rate), Gateway Out6/1
  Gateway Out5/1 -> Mod Ctrl/6  "IQ Sel"
  Delay2/1 -> Gateway Out3/1
  Gateway Out6/1 -> Mod Ctrl/7  "Full Rate Sym"
  Gateway Out7/1 -> Mod Ctrl/8  "Pilot I"
  Pilot Shift/1 -> Pilot Gen/3(Pilot Shift)

== system wlan_phy_tx_pmd/PSDU Syms Gen/Modulate/QPSK Mod ==
  b[1:0] : Inport
  Constant2 : xbsIndex_r4/Constant  const=Mod_Constellation_QPSK(1)  gui_display_data_type=Fixed-point  arith_type=Signed (2's comp)  n_bits=12  bin_pt=11  preci_type=Single  exp_width=8  frac_width=24  explicit_period=off  period=1  equ=P=C  opselect=C  inp2=PCIN>>17  opr=+  inp1=P  carry=CIN  dbl_ovrd=off  block_type=constant
  Constant3 : xbsIndex_r4/Constant  const=Mod_Constellation_QPSK(2)  gui_display_data_type=Fixed-point  arith_type=Signed (2's comp)  n_bits=12  bin_pt=11  preci_type=Single  exp_width=8  frac_width=24  explicit_period=off  period=1  equ=P=C  opselect=C  inp2=PCIN>>17  opr=+  inp1=P  carry=CIN  dbl_ovrd=off  block_type=constant
  LSB : xbsIndex_r4/Slice  nbits=1  boolean_output=off  mode=Lower Bit Location + Width  bit1=0  base1=MSB of Input  bit0=0  base0=LSB of Input  dbl_ovrd=off  block_type=slice
  LSB+1 : xbsIndex_r4/Slice  nbits=1  boolean_output=off  mode=Lower Bit Location + Width  bit1=0  base1=MSB of Input  bit0=1  base0=LSB of Input  dbl_ovrd=off  block_type=slice
  Mux : xbsIndex_r4/Mux  inputs=2  en=off  latency=0  precision=Full  arith_type=Unsigned  n_bits=16  bin_pt=14  quantization=Truncate  overflow=Wrap  dbl_ovrd=off  block_type=mux
  Mux1 : xbsIndex_r4/Mux  inputs=2  en=off  latency=0  precision=Full  arith_type=Unsigned  n_bits=16  bin_pt=14  quantization=Truncate  overflow=Wrap  dbl_ovrd=off  block_type=mux
  I : Outport
  Q : Outport  Port=2
  wires:
  Mux1/1 -> Q/1
  Mux/1 -> I/1
  Constant3/1 -> Mux1/3, Mux/3
  Constant2/1 -> Mux1/2, Mux/2
  b[1:0]/1 -> LSB/1, LSB+1/1
  LSB/1 -> Mux/1
  LSB+1/1 -> Mux1/1

== system wlan_phy_tx_pmd/PSDU Syms Gen/Pkt Data/BRAM IF 64b ==
  note: BRAM_Addr is a UFix32_0 value interpretted as a byte address by
      | the BRAM block. The BRAM is a 64-bit memory and requires BRAM_Addr
      | to be aligned for 64-bit accesses. Thus the 3LSB of the BRAM_Addr
      | signal must always be 0.
      |
      | In the current ref design the Tx Pkt Buf BRAM is 32KB (2^15 bytes),
      | divided into 8 4KB packet buffers.
      |
      | The Tx PHY Byte Address is 12 bits (4KB addressable). The 3 LSB are
      | trimmed to construct the 64-bit-word address.
      |
      | The Tx_PKT_BUF_SEL signal is 4 bits, but only takes values 0:7.
      |
      | Pkt_Buf_Addr_Offset is a software-programmed value which defines
      | the "0" address in the BRAM from the PHY's perspective. This offset
      | allows software to store meta data in the pkt buffer before the actual pkt
      | payload. The PHY's zero-address starts at that offset.
  Byte Addr : Inport
  12 LSB : xbsIndex_r4/Slice  nbits=ceil(log2(MAX_NUM_BYTES))  boolean_output=off  mode=Lower Bit Location + Width  bit1=0  base1=MSB of Input  bit0=0  base0=LSB of Input  dbl_ovrd=off  block_type=slice
      settings: block_version=8.2.02
  3 LSB : xbsIndex_r4/Slice  nbits=3  boolean_output=off  mode=Lower Bit Location + Width  bit1=0  base1=MSB of Input  bit0=0  base0=LSB of Input  dbl_ovrd=off  block_type=slice
      settings: block_version=8.2.02
  AddSub : xbsIndex_r4/AddSub  mode=Addition  use_carryin=off  use_carryout=off  en=off  latency=0  precision=User Defined  arith_type=Unsigned  n_bits=ceil(log2(MAX_NUM_BYTES))-3  bin_pt=0  quantization=Truncate  overflow=Wrap  dbl_ovrd=off  use_behavioral_HDL=off  hw_selection=Fabric  pipelined=off  block_type=addsub
  BRAM Addr Map : Subsystem
  BRAM Interface : Subsystem
  Byte Sel : Subsystem
  Delay4 : xbsIndex_r4/Delay  rst=off  infoeditControl=Selection of Reset will increase slice count due to use of real FFs and instead of SRLs  en=off  latency=1  dbl_ovrd=off  reg_retiming=off  block_type=delay
  Display : Display
  Gateway Out3 : xbsIndex_r4/Gateway Out  inherit_from_input=off  hdl_port=off  timing_constraint=None  locs_specified=off  LOCs={}  UseAsDAC=off  DACChannel='1'  block_type=gatewayout
  N MSB : xbsIndex_r4/Slice  nbits=ceil(log2(MAX_NUM_BYTES))-3  boolean_output=off  mode=Upper Bit Location + Width  bit1=0  base1=MSB of Input  bit0=0  base0=LSB of Input  dbl_ovrd=off  block_type=slice
      settings: block_version=8.2.02
  RAM Byte : Outport
  wires:
  BRAM Addr Map/1(Mem Addr) -> N MSB/1, 3 LSB/1
  [Tx_PKT_BUF_SEL] -> BRAM Interface/1(Pkt Buf Index)
  N MSB/1 -> AddSub/2
  [regTx_Pkt_Buf_Addr_Offset] -> AddSub/1, Gateway Out3/1
  Byte Addr/1 -> 12 LSB/1
  AddSub/1 -> BRAM Interface/2(64b Word Addr)
  BRAM Interface/1(64b Data) -> Byte Sel/1(64b)
  3 LSB/1 -> Delay4/1
  Byte Sel/1(B) -> RAM Byte/1
  12 LSB/1 -> BRAM Addr Map/1(Tx Ind)
  Delay4/1 -> Byte Sel/2(B Sel)
  Gateway Out3/1 -> Display/1

== system wlan_phy_tx_pmd/PSDU Syms Gen/Pkt Data/Bit Select ==
  b Sel : Inport
  B : Inport  Port=2
  Mux : xbsIndex_r4/Mux  inputs=8  en=off  latency=0  precision=Full  arith_type=Unsigned  n_bits=16  bin_pt=14  quantization=Truncate  overflow=Wrap  dbl_ovrd=off  block_type=mux
  b0 : xbsIndex_r4/Slice  nbits=1  boolean_output=off  mode=Lower Bit Location + Width  bit1=0  base1=MSB of Input  bit0=0  base0=LSB of Input  dbl_ovrd=off  block_type=slice
  b1 : xbsIndex_r4/Slice  nbits=1  boolean_output=off  mode=Lower Bit Location + Width  bit1=0  base1=MSB of Input  bit0=1  base0=LSB of Input  dbl_ovrd=off  block_type=slice
  b2 : xbsIndex_r4/Slice  nbits=1  boolean_output=off  mode=Lower Bit Location + Width  bit1=0  base1=MSB of Input  bit0=2  base0=LSB of Input  dbl_ovrd=off  block_type=slice
  b3 : xbsIndex_r4/Slice  nbits=1  boolean_output=off  mode=Lower Bit Location + Width  bit1=0  base1=MSB of Input  bit0=3  base0=LSB of Input  dbl_ovrd=off  block_type=slice
  b4 : xbsIndex_r4/Slice  nbits=1  boolean_output=off  mode=Lower Bit Location + Width  bit1=0  base1=MSB of Input  bit0=4  base0=LSB of Input  dbl_ovrd=off  block_type=slice
  b5 : xbsIndex_r4/Slice  nbits=1  boolean_output=off  mode=Lower Bit Location + Width  bit1=0  base1=MSB of Input  bit0=5  base0=LSB of Input  dbl_ovrd=off  block_type=slice
  b6 : xbsIndex_r4/Slice  nbits=1  boolean_output=off  mode=Lower Bit Location + Width  bit1=0  base1=MSB of Input  bit0=6  base0=LSB of Input  dbl_ovrd=off  block_type=slice
  b7 : xbsIndex_r4/Slice  nbits=1  boolean_output=off  mode=Lower Bit Location + Width  bit1=0  base1=MSB of Input  bit0=7  base0=LSB of Input  dbl_ovrd=off  block_type=slice
  b : Outport
  wires:
  Mux/1 -> b/1
  B/1 -> b7/1, b6/1, b5/1, b4/1, b3/1, b2/1, b1/1, b0/1
  b0/1 -> Mux/2
  b1/1 -> Mux/3
  b2/1 -> Mux/4
  b3/1 -> Mux/5
  b4/1 -> Mux/6
  b5/1 -> Mux/7
  b6/1 -> Mux/8
  b7/1 -> Mux/9
  b Sel/1 -> Mux/1

== system wlan_phy_tx_pmd/PSDU Syms Gen/Pkt Data/Byte Src Sel ==
  Sel Zero : Inport
  Sel FCS : Inport  Port=2
  "Sel HTSIG " : Inport  Port=3
  Data B : Inport  Port=4
  FCS B : Inport  Port=5
  HTSIG : Inport  Port=6
  Byte Select : Scope  NumInputPorts=7
      settings: YMin=-5~-5~-5~-5~-5~-5~-5  YMax=5~5~5~5~5~5~5  SaveName=ScopeData7
  Concat : xbsIndex_r4/Concat  num_inputs=2  dbl_ovrd=off  block_type=concat
  Constant1 : xbsIndex_r4/Constant  const=0  gui_display_data_type=Fixed-point  arith_type=Unsigned  n_bits=8  bin_pt=0  preci_type=Single  exp_width=8  frac_width=24  explicit_period=off  period=1  equ=P=C  opselect=C  inp2=PCIN>>17  opr=+  inp1=P  carry=CIN  dbl_ovrd=off  block_type=constant
  Constant2 : xbsIndex_r4/Constant  const=0  gui_display_data_type=Fixed-point  arith_type=Unsigned  n_bits=8  bin_pt=0  preci_type=Single  exp_width=8  frac_width=24  explicit_period=off  period=1  equ=P=C  opselect=C  inp2=PCIN>>17  opr=+  inp1=P  carry=CIN  dbl_ovrd=off  block_type=constant
  Gateway Out{1..6,9} (7 alike) : xbsIndex_r4/Gateway Out  inherit_from_input=off  hdl_port=off  timing_constraint=None  locs_specified=off  LOCs={}  UseAsDAC=off  DACChannel='1'  block_type=gatewayout
  Mux : xbsIndex_r4/Mux  inputs=4  en=off  latency=0  precision=Full  arith_type=Unsigned  n_bits=16  bin_pt=14  quantization=Truncate  overflow=Wrap  dbl_ovrd=off  block_type=mux
  Mux1 : xbsIndex_r4/Mux  inputs=2  en=off  latency=0  precision=Full  arith_type=Unsigned  n_bits=16  bin_pt=14  quantization=Truncate  overflow=Wrap  dbl_ovrd=off  block_type=mux
  Tx Byte : Outport
  wires:
  Concat/1 -> Mux/1
  Sel FCS/1 -> Concat/2, Gateway Out1/1
  Data B/1 -> Mux/2, Gateway Out2/1
  "Sel HTSIG "/1 -> Concat/1, Gateway Out4/1
  FCS B/1 -> Mux/3, Gateway Out3/1
  Mux/1 -> Mux1/2
  Gateway Out9/1 -> Byte Select/1  "Sel Zero"
  Gateway Out1/1 -> Byte Select/2  "Sel FCS"
  Gateway Out2/1 -> Byte Select/4  "Data Byte"
  Gateway Out3/1 -> Byte Select/5  "FCS Byte"
  Sel Zero/1 -> Mux1/1, Gateway Out9/1
  Constant1/1 -> Mux1/3
  Mux1/1 -> Tx Byte/1, Gateway Out6/1
  HTSIG/1 -> Mux/4, Gateway Out5/1
  Constant2/1 -> Mux/5
  Gateway Out4/1 -> Byte Select/3  "Sel HTSIG"
  Gateway Out5/1 -> Byte Select/6  "HTSIG Byte"
  Gateway Out6/1 -> Byte Select/7  "Tx Byte"

== system wlan_phy_tx_pmd/PSDU Syms Gen/Pkt Data/FCS Calc ==
  note: FCS covers bytes starting with first MAC payload byte.
      | For 11ag FCS starts after SIGNAL (3B) and SERVICE (2B).
      | For 11n FCS starts after L-SIG (3B), HT-SIG (6B) and SERVICE (2B).
  note: Checksum bytes must be output [0,1,2,3], even when they're
      | not aligned to a 32-bit boundary in the actual payload. The
      | CRC bytes are selected [0,1,2,3] here, adjusting the 2 LSB
      | of the actual byte index to count from 0 during the FCS output.
  note: Don't udpate CRC state while checksum
      | is being read by Tx pipeline
  FCS Sel : Inport
  Byte : Inport  Port=2
  Byte Ind : Inport  Port=3
  Byte Valid : Inport  Port=4
  2LSB : xbsIndex_r4/Slice  nbits=2  boolean_output=off  mode=Lower Bit Location + Width  bit1=0  base1=MSB of Input  bit0=0  base0=LSB of Input  dbl_ovrd=off  block_type=slice
  AddSub : xbsIndex_r4/AddSub  mode=Subtraction  use_carryin=off  use_carryout=off  en=off  latency=0  precision=User Defined  arith_type=Unsigned  n_bits=2  bin_pt=0  quantization=Truncate  overflow=Wrap  dbl_ovrd=off  use_behavioral_HDL=off  hw_selection=Fabric  pipelined=off  block_type=addsub
  Byte Sel : Subsystem
  CRC32 Calc : Subsystem
  Constant2 : xbsIndex_r4/Constant  const=5  gui_display_data_type=Fixed-point  arith_type=Unsigned  n_bits=3  bin_pt=0  preci_type=Single  exp_width=8  frac_width=24  explicit_period=off  period=1  equ=P=C  opselect=C  inp2=PCIN>>17  opr=+  inp1=P  carry=CIN  dbl_ovrd=off  block_type=constant
  Constant3 : xbsIndex_r4/Constant  const=11  gui_display_data_type=Fixed-point  arith_type=Unsigned  n_bits=4  bin_pt=0  preci_type=Single  exp_width=8  frac_width=24  explicit_period=off  period=1  equ=P=C  opselect=C  inp2=PCIN>>17  opr=+  inp1=P  carry=CIN  dbl_ovrd=off  block_type=constant
  FCS Calc : Scope  NumInputPorts=7
      settings: TimeRange=12000  YMin=0~0~0~0~0~0~-1  YMax=70~1~1~1~3~300~1  SaveName=ScopeData5
  Gateway Out{1..6} (6 alike) : xbsIndex_r4/Gateway Out  inherit_from_input=off  hdl_port=off  timing_constraint=None  locs_specified=off  LOCs={}  UseAsDAC=off  DACChannel='1'  block_type=gatewayout
  Inverter : xbsIndex_r4/Inverter  en=off  latency=0  dbl_ovrd=off  block_type=inv
  Logical1 : xbsIndex_r4/Logical  logical_function=OR  inputs=2  en=off  latency=0  precision=Full  arith_type=Unsigned  n_bits=16  bin_pt=0  align_bp=on  dbl_ovrd=off  block_type=logical
  Logical2 : xbsIndex_r4/Logical  logical_function=AND  inputs=3  en=off  latency=0  precision=Full  arith_type=Unsigned  n_bits=16  bin_pt=0  align_bp=on  dbl_ovrd=off  block_type=logical
  Logical3 : xbsIndex_r4/Logical  logical_function=AND  inputs=2  en=off  latency=0  precision=Full  arith_type=Unsigned  n_bits=16  bin_pt=0  align_bp=on  dbl_ovrd=off  block_type=logical
  Logical5 : xbsIndex_r4/Logical  logical_function=AND  inputs=3  en=off  latency=0  precision=Full  arith_type=Unsigned  n_bits=16  bin_pt=0  align_bp=on  dbl_ovrd=off  block_type=logical
  Register : xbsIndex_r4/Register  init=0  rst=on  en=on  dbl_ovrd=off  block_type=register
  Relational1 : xbsIndex_r4/Relational  mode=a>=b  en=off  latency=0  dbl_ovrd=off  block_type=relational
  Relational2 : xbsIndex_r4/Relational  mode=a>=b  en=off  latency=0  dbl_ovrd=off  block_type=relational
  posedge : Subsystem
  CRC Byte : Outport
  wires:
  Byte Sel/1(B) -> CRC Byte/1, Gateway Out6/1
  Byte/1 -> CRC32 Calc/1(byte)
  CRC32 Calc/1(CRC32) -> Byte Sel/1(32b)
  Relational2/1 -> Logical2/3
  Constant2/1 -> Relational2/2
  Byte Ind/1 -> Relational2/1, Gateway Out3/1, Relational1/1, 2LSB/1
  Byte Valid/1 -> Logical2/2, Logical5/2, Gateway Out1/1
  [Tx_PHY_Mode_11ag] -> Logical2/1
  Relational1/1 -> Logical5/3
  Constant3/1 -> Relational1/2
  [Tx_PHY_Mode_11n] -> Logical5/1
  Logical2/1 -> Logical1/1
  Logical5/1 -> Logical1/2
  Gateway Out1/1 -> FCS Calc/2  "Byte Ind Valid"
  Gateway Out3/1 -> FCS Calc/1  "Byte Ind"
  Gateway Out2/1 -> FCS Calc/3  "FCS Sel"
  Gateway Out4/1 -> FCS Calc/4  "CRC32 En"
  Gateway Out5/1 -> FCS Calc/5  "FCS B Sel"
  Logical3/1 -> CRC32 Calc/2(en), Gateway Out4/1
  Logical1/1 -> Logical3/1
  AddSub/1 -> Gateway Out5/1, Byte Sel/2(B Sel)
  Gateway Out6/1 -> FCS Calc/6  "FCS Byte"
  FCS Sel/1 -> Inverter/1, Gateway Out2/1, posedge/1(D)
  Inverter/1 -> Logical3/2
  2LSB/1 -> Register/1, AddSub/2
  posedge/1(Q) -> Register/3
  [TX_RESET] -> Register/2
  Register/1 -> AddSub/1
